simulink model "sldvmiscovtool_sample"  (Simulink 6.6)
settings: Solver=FixedStepDiscrete  StartTime=0.0  StopTime=50  FixedStep=0.01  RelTol=1e-3
undefined symbols (not defined in the file or in its folder): DiscIntNeverNeededParam
libraries: sldvlib x1
Description:
  | Cruise Control Test Generation Example
settings Model: Creator=The MathWorks Inc.  LastModifiedBy=yito  CovMetricSettings=dcme  CovHtmlReporting=off  covSaveCumulativeToWorkspaceVar=off  CovSaveSingleToWorkspaceVar=off  ExtModeAutoUpdateStatusClock=off
settings OptimizationCC: InlineParams=on  InlineInvariantSignals=on
settings DebuggingCC: SignalResolutionControl=TryResolveAllWithWarning
settings HardwareCC: TargetHWDeviceType=32-bit Generic
settings ConfigComp: Description=Design Verifier Custom Configuration Component  DVMaxProcessTime=600  DVDisplayUnsatisfiableObjectives=on  DVMakeOutputFilesUnique=off  DVModelCoverageObjectives=MCDC  DVMaxTestCaseSteps=500  DVTestSuiteOptimization=CombinedObjectives  DVAssertions=EnableAll  DVProofAssumptions=EnableAll  DVProvingStrategy=FindViolation  DVSaveHarnessModel=on  DVSaveReport=on  DVDisplayReport=off

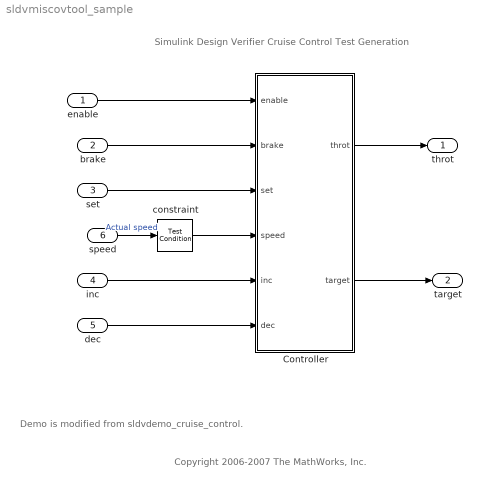
== system sldvmiscovtool_sample ==
  note: Simulink Design Verifier
      | Cruise Control Test Generation
  note: Copyright 2006-2007 The MathWorks, Inc.
  note: Demo is modified from sldvdemo_cruise_control.
  enable : Inport  DataType=boolean  Interpolate=off
  brake : Inport  Port=2  DataType=boolean  Interpolate=off
  set : Inport  Port=3  DataType=boolean  Interpolate=off
  inc : Inport  Port=4  DataType=boolean  Interpolate=off
  dec : Inport  Port=5  DataType=boolean  Interpolate=off
  speed : Inport  Port=6  DataType=double  Interpolate=off
  Controller : Subsystem
  constraint : sldvlib/Test Condition  SystemSampleTime=-1  enabled=on  customAVTBlockType=Test Condition  intervals=[0 100]  initial=off  dispValues=on  outEnabled=on
      settings: AttributesFormatString=%<intervals>
  throt : Outport
  target : Outport  Port=2
  wires:
  enable/1 -> Controller/1(enable)
  brake/1 -> Controller/2(brake)
  set/1 -> Controller/3(set)
  Controller/1(throt) -> throt/1
  inc/1 -> Controller/5(inc)
  dec/1 -> Controller/6(dec)
  Controller/2(target) -> target/1
  speed/1 -> constraint/1  "Actual speed"
  constraint/1 -> Controller/4(speed)

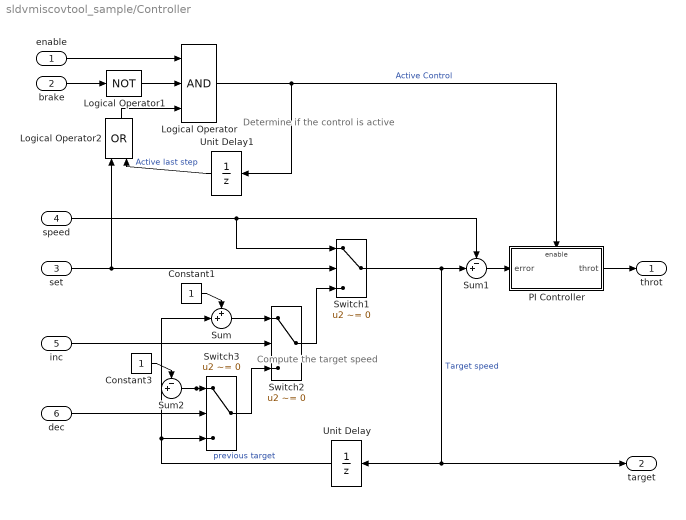
== system sldvmiscovtool_sample/Controller ==
  note: Determine if the
      | control is active
  note: Compute the
      | target speed
  enable : Inport  DataType=boolean
  brake : Inport  Port=2  DataType=boolean
  set : Inport  Port=3  DataType=boolean
  speed : Inport  Port=4  DataType=double
  inc : Inport  Port=5  DataType=boolean
  dec : Inport  Port=6  DataType=boolean
  Constant1 : Constant
  Constant3 : Constant
  Logical Operator : Logic  Inputs=3  AllPortsSameDT=off  OutDataTypeMode=Boolean
  Logical Operator1 : Logic  Operator=NOT  AllPortsSameDT=off  OutDataTypeMode=Boolean
  Logical Operator2 : Logic  Orientation=up  Operator=OR  AllPortsSameDT=off  OutDataTypeMode=Boolean
  PI Controller : Subsystem
  Sum : Sum  Inputs=++|
  Sum1 : Sum  Inputs=-+|
  Sum2 : Sum  Inputs=-+|
  Switch1 : Switch  Criteria=u2 ~= 0
  Switch2 : Switch  Criteria=u2 ~= 0
  Switch3 : Switch  Criteria=u2 ~= 0
  Unit Delay : UnitDelay  Orientation=left  SampleTime=0.01
  Unit Delay1 : UnitDelay  Orientation=left  SampleTime=0.01
  throt : Outport
  target : Outport  Port=2
  wires:
  brake/1 -> Logical Operator1/1
  enable/1 -> Logical Operator/1
  Logical Operator1/1 -> Logical Operator/2
  set/1 -> Switch1/2, Logical Operator2/1
  speed/1 -> Sum1/1, Switch1/1
  inc/1 -> Switch2/2
  Constant1/1 -> Sum/1
  Sum/1 -> Switch2/1
  dec/1 -> Switch3/2
  Constant3/1 -> Sum2/1
  Sum2/1 -> Switch3/1
  Switch2/1 -> Switch1/3
  Switch3/1 -> Switch2/3
  Unit Delay/1 -> Sum/2, Sum2/2, Switch3/3  "previous target"
  Switch1/1 -> Unit Delay/1, target/1, Sum1/2  "Target speed"
  Logical Operator2/1 -> Logical Operator/3
  Unit Delay1/1 -> Logical Operator2/2  "Active last step"
  Logical Operator/1 -> Unit Delay1/1, PI Controller/Enable  "Active Control"
  Sum1/1 -> PI Controller/1(error)
  PI Controller/1(throt) -> throt/1

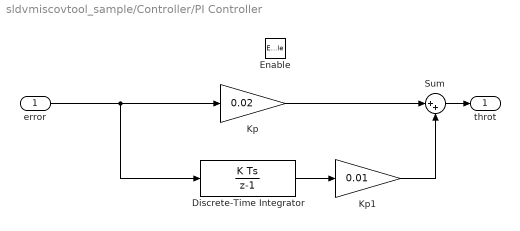
== system sldvmiscovtool_sample/Controller/PI Controller ==
  error : Inport
  Enable : EnablePort
  Discrete-Time Integrator : DiscreteIntegrator  SampleTime=0.01  LimitOutput=on  UpperSaturationLimit=5  LowerSaturationLimit=-5  ICPrevOutput=DiscIntNeverNeededParam  ICPrevScaledInput=DiscIntNeverNeededParam
  Kp : Gain  Gain=0.02
  Kp1 : Gain  Gain=0.01
  Sum : Sum  Inputs=|++
  throt : Outport
  wires:
  Kp/1 -> Sum/1
  Kp1/1 -> Sum/2
  Discrete-Time Integrator/1 -> Kp1/1
  error/1 -> Kp/1, Discrete-Time Integrator/1
  Sum/1 -> throt/1
